simulink model "Dynamics_test2_sim"  (R2016b)
settings: Solver=VariableStepAuto  StartTime=0.0  StopTime=1000  FixedStep=1  RelTol=1e-3
values from neighbouring files (symbols this model uses):
  fsw_params = init_fsw_params()    [init_dynamics_test_new.m]
  MT_dipole_const = 0.15*ones(3,1)    [init_dynamics_test_new.m]
  MT_input = 1    [init_dynamics_test_new.m]
  RW_input = 1    [init_dynamics_test_new.m]
  RW_torque_const = [0;0;0]    [init_dynamics_test_new.m]
  sim_params = struct('CAN',sim_params.CAN,'dynamics',dynamics,'sensors',sim_params.sensors,'actuators',sim_params.actuators,'environment',sim_params.environment,'bus',sim_params.bus)    [Dynamics_test.m]
undefined symbols (not defined in the file or in its folder): disturbances_lib, DT_aero_eci_Nm, DT_dipole_body_Am2, DT_grav_eci_Nm, DT_solar_eci_Nm, env_acc_eci_mps2, Environment, environment_lib, GPS_time, init_pos_eci_km, init_vel_eci_kmps, mag_vec_eci, sun_vec_eci
libraries: bus_stubs_template x2, dynamics_lib x1, GPS_time_lib x1, aero_drag_lib x1, gravity_lib_2 x1, mag_vec_lib x1, solar_pressure_lib x1, sun_vector_lib x1, time_coord_rotation_lib x1, tle2eci_coarse_lib x1
settings Model: Creator=Ryan  LastModifiedBy=evich

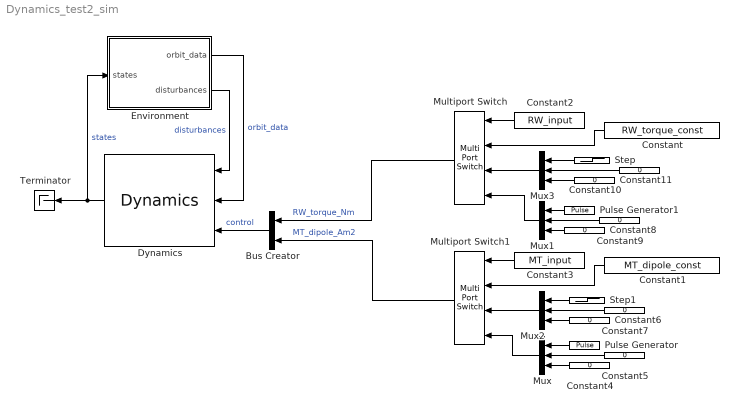
== system Dynamics_test2_sim ==
  Bus Creator : BusCreator  Inputs=2
  Constant : Constant  Value=RW_torque_const
  Constant1 : Constant  Value=MT_dipole_const
  Constant{4..11} (8 alike) : Constant  Value=0
  Constant2 : Constant  Value=RW_input
  Constant3 : Constant  Value=MT_input
  Dynamics : dynamics_lib/Dynamics
  Environment : Subsystem  AncestorBlock=environment_lib/Environment
  Multiport Switch : MultiPortSwitch  DiagnosticForDefault=Warning
  Multiport Switch1 : MultiPortSwitch  DiagnosticForDefault=Warning
  Mux{,1..3} (4 alike) : Mux  Inputs=3
  Pulse Generator : DiscretePulseGenerator  PulseType=Time based  Amplitude=0.15  Period=500  PulseWidth=0.1  PhaseDelay=200
  Pulse Generator1 : DiscretePulseGenerator  PulseType=Time based  Amplitude=fsw_params.control.pd_controller.max_torque  Period=500  PulseWidth=.1  PhaseDelay=200
  Step : Step  Before=fsw_params.control.pd_controller.max_torque  After=0  SampleTime=0
  Step1 : Step  Before=0.15  After=0  SampleTime=0
  Terminator : Terminator
  wires:
  Environment/2(disturbances) -> Dynamics/1  "disturbances"
  Environment/1(orbit_data) -> Dynamics/2  "orbit_data"
  Bus Creator/1 -> Dynamics/3  "control"
  Multiport Switch/1 -> Bus Creator/1  "RW_torque_Nm"
  Multiport Switch1/1 -> Bus Creator/2  "MT_dipole_Am2"
  Dynamics/1 -> Terminator/1, Environment/1(states)  "states"
  Constant2/1 -> Multiport Switch/1
  Constant/1 -> Multiport Switch/2
  Constant1/1 -> Multiport Switch1/2
  Constant3/1 -> Multiport Switch1/1
  Pulse Generator/1 -> Mux/1
  Mux/1 -> Multiport Switch1/4
  Constant4/1 -> Mux/3
  Constant5/1 -> Mux/2
  Mux2/1 -> Multiport Switch1/3
  Step1/1 -> Mux2/1
  Constant6/1 -> Mux2/3
  Constant7/1 -> Mux2/2
  Pulse Generator1/1 -> Mux1/1
  Mux1/1 -> Multiport Switch/4
  Constant8/1 -> Mux1/3
  Constant9/1 -> Mux1/2
  Mux3/1 -> Multiport Switch/3
  Step/1 -> Mux3/1
  Constant10/1 -> Mux3/3
  Constant11/1 -> Mux3/2

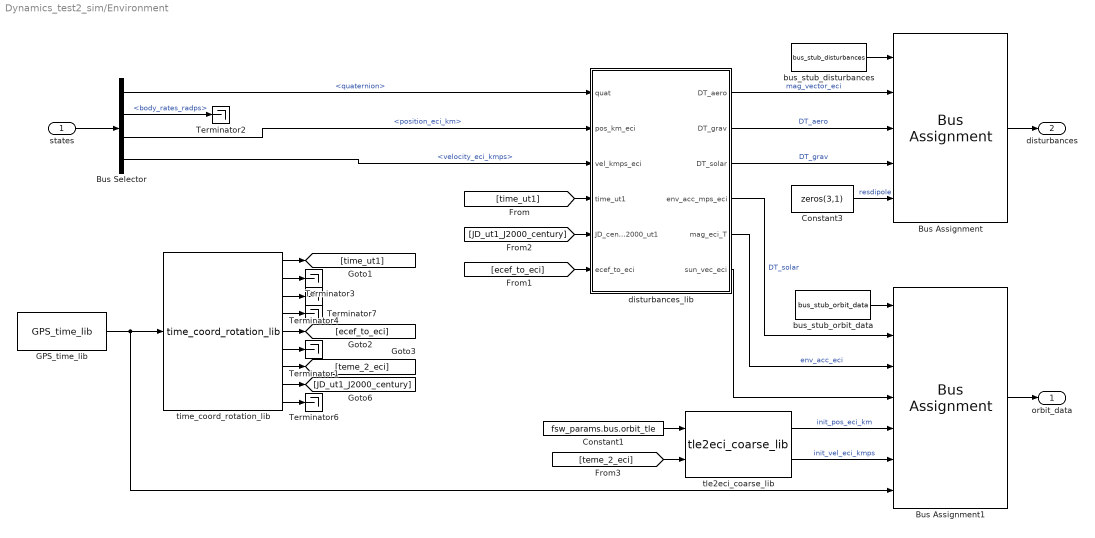
== system Dynamics_test2_sim/Environment ==
  states : Inport  OutDataTypeStr=Bus: states
  Bus Assignment : BusAssignment  AssignedSignals=DT_aero_eci_Nm,DT_grav_eci_Nm,DT_solar_eci_Nm,DT_dipole_body_Am2
  Bus Assignment1 : BusAssignment  AssignedSignals=env_acc_eci_mps2,mag_vec_eci,sun_vec_eci,init_pos_eci_km,init_vel_eci_kmps,GPS_time
  Bus Selector : BusSelector  OutputSignals=quaternion,body_rates_radps,position_eci_km,velocity_eci_kmps
  Constant1 : Constant  Value=fsw_params.bus.orbit_tle
  Constant3 : Constant  Value=zeros(3,1)
  GPS_time_lib : GPS_time_lib/GPS_time_lib
  Terminator{1..4,6..7} (6 alike) : Terminator
  bus_stub_disturbances : bus_stubs_template/bus_stub_disturbances
  bus_stub_orbit_data : bus_stubs_template/bus_stub_orbit_data
  disturbances_lib : Subsystem  AncestorBlock=disturbances_lib/disturbances_lib
  time_coord_rotation_lib : time_coord_rotation_lib/time_coord_rotation_lib
  tle2eci_coarse_lib : tle2eci_coarse_lib/tle2eci_coarse_lib
  orbit_data : Outport
  disturbances : Outport  Port=2
  wires:
  tle2eci_coarse_lib/2 -> Bus Assignment1/6  "init_vel_eci_kmps"
  tle2eci_coarse_lib/1 -> Bus Assignment1/5  "init_pos_eci_km"
  Constant1/1 -> tle2eci_coarse_lib/1
  bus_stub_disturbances/1 -> Bus Assignment/1
  Bus Assignment/1 -> disturbances/1
  states/1 -> Bus Selector/1
  Bus Selector/1 -> disturbances_lib/1(quat)  "<quaternion>"
  Bus Selector/2 -> Terminator2/1  "<body_rates_radps>"
  Bus Selector/3 -> disturbances_lib/2(pos_km_eci)  "<position_eci_km>"
  Bus Selector/4 -> disturbances_lib/3(vel_kmps_eci)  "<velocity_eci_kmps>"
  [time_ut1] -> disturbances_lib/4(time_ut1)
  Constant3/1 -> Bus Assignment/5  "resdipole"
  bus_stub_orbit_data/1 -> Bus Assignment1/1
  Bus Assignment1/1 -> orbit_data/1
  disturbances_lib/6(sun_vec_eci) -> Bus Assignment1/4
  [JD_ut1_J2000_century] -> disturbances_lib/5(JD_cent_J2000_ut1)
  [ecef_to_eci] -> disturbances_lib/6(ecef_to_eci)
  disturbances_lib/1(DT_aero) -> Bus Assignment/2  "mag_vector_eci"
  disturbances_lib/2(DT_grav) -> Bus Assignment/3  "DT_aero"
  disturbances_lib/3(DT_solar) -> Bus Assignment/4  "DT_grav"
  disturbances_lib/4(env_acc_mps_eci) -> Bus Assignment1/2  "DT_solar"
  disturbances_lib/5(mag_eci_T) -> Bus Assignment1/3  "env_acc_eci"
  GPS_time_lib/1 -> Bus Assignment1/7, time_coord_rotation_lib/1
  [teme_2_eci] -> tle2eci_coarse_lib/2
  time_coord_rotation_lib/1 -> [time_ut1]
  time_coord_rotation_lib/2 -> Terminator3/1
  time_coord_rotation_lib/3 -> Terminator4/1
  time_coord_rotation_lib/4 -> Terminator7/1
  time_coord_rotation_lib/5 -> [ecef_to_eci]
  time_coord_rotation_lib/9 -> Terminator6/1
  time_coord_rotation_lib/8 -> [JD_ut1_J2000_century]
  time_coord_rotation_lib/7 -> [teme_2_eci]
  time_coord_rotation_lib/6 -> Terminator1/1

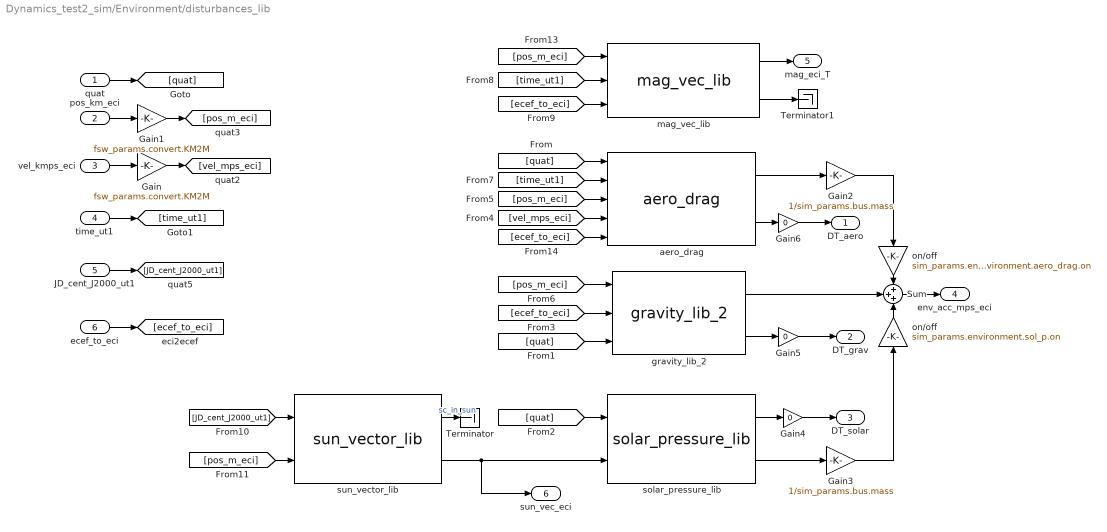
== system Dynamics_test2_sim/Environment/disturbances_lib ==
  quat : Inport
  pos_km_eci : Inport  Port=2
  vel_kmps_eci : Inport  Port=3
  time_ut1 : Inport  Port=4
  JD_cent_J2000_ut1 : Inport  Port=5
  ecef_to_eci : Inport  Port=6
  Gain : Gain  Gain=fsw_params.convert.KM2M
  Gain1 : Gain  Gain=fsw_params.convert.KM2M
  Gain2 : Gain  Gain=1/sim_params.bus.mass
  Gain3 : Gain  Gain=1/sim_params.bus.mass
  Gain4 : Gain  Gain=0
  Gain5 : Gain  Gain=0
  Gain6 : Gain  Gain=0
  Sum : Sum  Inputs=+++
  Terminator : Terminator
  Terminator1 : Terminator
  aero_drag : aero_drag_lib/aero_drag
  gravity_lib_2 : gravity_lib_2/gravity_lib_2
  mag_vec_lib : mag_vec_lib/mag_vec_lib
  on/off : Gain  Gain=sim_params.environment.aero_drag.on
  "on/off " : Gain  Gain=sim_params.environment.sol_p.on
  solar_pressure_lib : solar_pressure_lib/solar_pressure_lib
  sun_vector_lib : sun_vector_lib/sun_vector_lib
  DT_aero : Outport
  DT_grav : Outport  Port=2
  DT_solar : Outport  Port=3
  env_acc_mps_eci : Outport  Port=4
  mag_eci_T : Outport  Port=5
  sun_vec_eci : Outport  Port=6
  wires:
  [ecef_to_eci] -> aero_drag/5
  quat/1 -> [quat]
  ecef_to_eci/1 -> [ecef_to_eci]
  [quat] -> aero_drag/1
  [quat] -> solar_pressure_lib/1
  [ecef_to_eci] -> gravity_lib_2/2
  vel_kmps_eci/1 -> Gain/1
  Gain/1 -> [vel_mps_eci]
  [vel_mps_eci] -> aero_drag/4
  pos_km_eci/1 -> Gain1/1
  Gain1/1 -> [pos_m_eci]
  [pos_m_eci] -> aero_drag/3
  [pos_m_eci] -> gravity_lib_2/1
  time_ut1/1 -> [time_ut1]
  [time_ut1] -> aero_drag/2
  [time_ut1] -> mag_vec_lib/2
  JD_cent_J2000_ut1/1 -> [JD_cent_J2000_ut1]
  [JD_cent_J2000_ut1] -> sun_vector_lib/1
  [pos_m_eci] -> sun_vector_lib/2
  sun_vector_lib/1 -> Terminator/1  "sc_in_sun"
  sun_vector_lib/2 -> sun_vec_eci/1, solar_pressure_lib/2
  [pos_m_eci] -> mag_vec_lib/1
  mag_vec_lib/2 -> Terminator1/1
  mag_vec_lib/1 -> mag_eci_T/1
  gravity_lib_2/1 -> Sum/2
  aero_drag/1 -> Gain2/1
  Gain2/1 -> on/off/1
  solar_pressure_lib/2 -> Gain3/1
  Gain3/1 -> "on/off "/1
  [ecef_to_eci] -> mag_vec_lib/3
  aero_drag/2 -> Gain6/1
  gravity_lib_2/2 -> Gain5/1
  solar_pressure_lib/1 -> Gain4/1
  Sum/1 -> env_acc_mps_eci/1
  on/off/1 -> Sum/1
  "on/off "/1 -> Sum/3
  [quat] -> gravity_lib_2/3
  Gain4/1 -> DT_solar/1
  Gain5/1 -> DT_grav/1
  Gain6/1 -> DT_aero/1
